simulink model "diagrama"  (R2013a)
settings: Solver=ode45  StartTime=0.0  StopTime=10.0  RelTol=1e-3
settings Model: Creator=mario  LastModifiedBy=mario

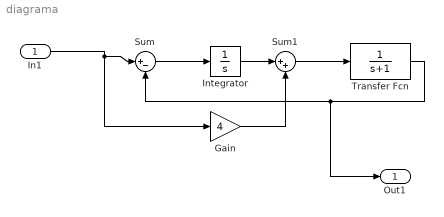
== system diagrama ==
  In1 : Inport
  Gain : Gain  Gain=4
  Integrator : Integrator
  Sum : Sum  Inputs=|+-
  Sum1 : Sum  Inputs=|++
  Transfer Fcn : TransferFcn  Denominator=[1 1]
  Out1 : Outport
  wires:
  In1/1 -> Gain/1, Sum/1
  Sum/1 -> Integrator/1
  Integrator/1 -> Sum1/1
  Sum1/1 -> Transfer Fcn/1
  Gain/1 -> Sum1/2
  Transfer Fcn/1 -> Out1/1, Sum/2
